simulink model "lab7_t27"  (R2021a)
settings: Solver=VariableStepAuto  StartTime=0.0  StopTime=10.0  RelTol=1e-3
settings Model: Creator=reemb  LastModifiedBy=reemb

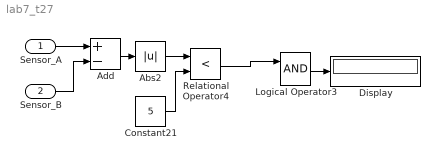
== system lab7_t27 ==
  Sensor_A : Inport
  Sensor_B : Inport  Port=2
  Abs2 : Abs
  Add : Sum  Inputs=+-
  Constant21 : Constant  Value=5
  Display : Display
  Logical Operator3 : Logic  AllPortsSameDT=off  OutDataTypeStr=boolean
  Relational Operator4 : RelationalOperator  Operator=<  OutDataTypeStr=boolean  RndMeth=Simplest
  wires:
  Relational Operator4/1 -> Logical Operator3/1
  Abs2/1 -> Relational Operator4/1
  Constant21/1 -> Relational Operator4/2
  Add/1 -> Abs2/1
  Sensor_A/1 -> Add/1
  Sensor_B/1 -> Add/2
  Logical Operator3/1 -> Display/1
